simulink model "System3"  (R2018b)
settings: Solver=VariableStepAuto  StartTime=0.0  StopTime=20  RelTol=1e-3
libraries: cstblocks x2
settings Model: Creator=Abraham Pérez  LastModifiedBy=Abraham Pérez

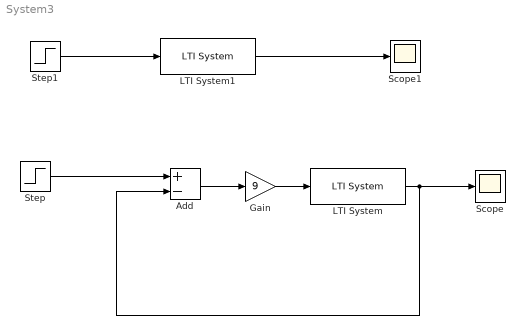
== system System3 ==
  Add : Sum  Inputs=+-
  Gain : Gain  Gain=9
  LTI System : cstblocks/LTI System  sys=g3  IC=[]
  LTI System1 : cstblocks/LTI System  sys=g3_  IC=[]
  Scope : Scope
  Scope1 : Scope
  Step : Step  SampleTime=0
  Step1 : Step  SampleTime=0
  wires:
  LTI System/1 -> Scope/1, Add/2
  LTI System1/1 -> Scope1/1
  Step1/1 -> LTI System1/1
  Gain/1 -> LTI System/1
  Add/1 -> Gain/1
  Step/1 -> Add/1
